simulink model "PrimRes_sharing"  (R2018a)
settings: Solver=VariableStepAuto  StartTime=0.0  StopTime=25  MaxStep=0.01  RelTol=1e-3
values from neighbouring files (symbols this model uses):
  Fn = 50    [PrimRes_sharing_Script.m]    (also in PrimRes_sharing_eigen_Script.m; PrimRes_sharing_steps_1_2MW_Script.m; PrimRes_sharing_steps_6MW_Script.m)
  KESS = Kess(4)    [PrimRes_sharing_Script.m]    (also in PrimRes_sharing_eigen_Script.m = Kess(i); PrimRes_sharing_steps_1_2MW_Script.m = Kess(i); PrimRes_sharing_steps_6MW_Script.m = Kess(i))
  KGT = Kgt(4)    [PrimRes_sharing_Script.m]    (also in PrimRes_sharing_eigen_Script.m = Kgt(i); PrimRes_sharing_steps_1_2MW_Script.m = Kgt(i); PrimRes_sharing_steps_6MW_Script.m = Kgt(i))
  Pessmax = 3    [PrimRes_sharing_Script.m]    (also in PrimRes_sharing_eigen_Script.m; PrimRes_sharing_steps_1_2MW_Script.m; PrimRes_sharing_steps_6MW_Script.m)
  Sn = 88    [PrimRes_sharing_Script.m]    (also in PrimRes_sharing_eigen_Script.m; PrimRes_sharing_steps_1_2MW_Script.m; PrimRes_sharing_steps_6MW_Script.m)
  StepMW = 6    [PrimRes_sharing_Script.m]    (also in PrimRes_sharing_eigen_Script.m = 1.2; PrimRes_sharing_steps_1_2MW_Script.m = 1.2; PrimRes_sharing_steps_6MW_Script.m)
  Tess = 0.05    [PrimRes_sharing_Script.m]    (also in PrimRes_sharing_eigen_Script.m; PrimRes_sharing_steps_1_2MW_Script.m; PrimRes_sharing_steps_6MW_Script.m)
  Tgov1 = 0.1    [PrimRes_sharing_Script.m]    (also in PrimRes_sharing_eigen_Script.m; PrimRes_sharing_steps_1_2MW_Script.m; PrimRes_sharing_steps_6MW_Script.m)
  Tgov2 = 0.4    [PrimRes_sharing_Script.m]    (also in PrimRes_sharing_eigen_Script.m; PrimRes_sharing_steps_1_2MW_Script.m; PrimRes_sharing_steps_6MW_Script.m)
settings Model: Creator=daniemot  LastModifiedBy=daniemot

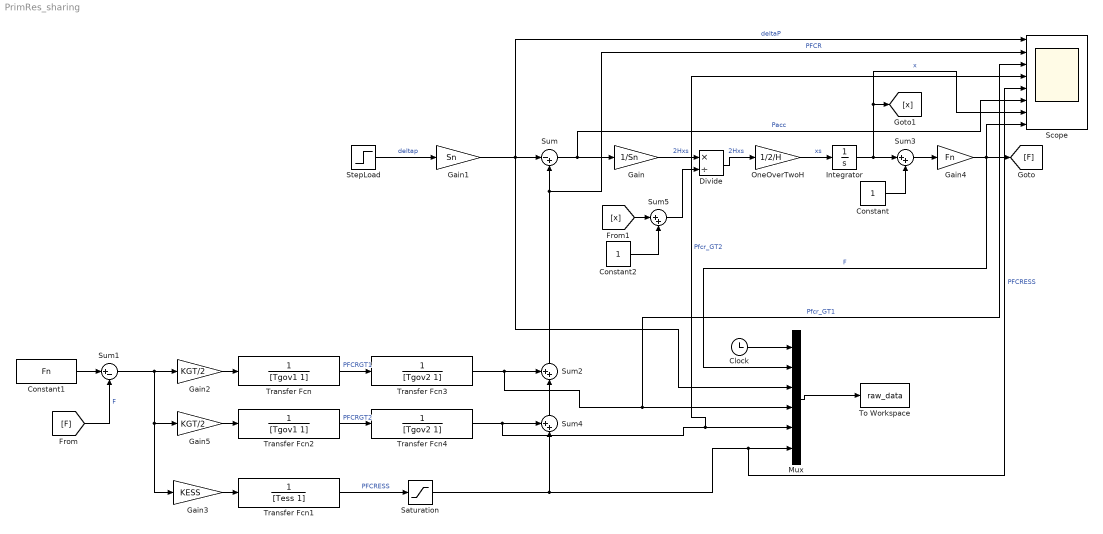
== system PrimRes_sharing ==
  Clock : Clock
  Constant : Constant
  Constant1 : Constant  Value=Fn
  Constant2 : Constant
  Divide : Product  Inputs=*/
  Gain : Gain  Gain=1/Sn
  Gain1 : Gain  Gain=Sn
  Gain2 : Gain  Gain=KGT/2
  Gain3 : Gain  Gain=KESS
  Gain4 : Gain  Gain=Fn
  Gain5 : Gain  Gain=KGT/2
  Integrator : Integrator
  Mux : Mux  Inputs=6
  OneOverTwoH : Gain  Gain=1/2/H
  Saturation : Saturate  UpperLimit=Pessmax  LowerLimit=-Pessmax
  Scope : Scope  NumInputPorts=8
  StepLoad : Step  After=StepMW/Sn  SampleTime=0
  Sum : Sum  Inputs=|-+
  Sum1 : Sum  Inputs=|+-
  Sum2 : Sum  Inputs=++|
  Sum3 : Sum  Inputs=|++
  Sum4 : Sum  Inputs=++|
  Sum5 : Sum  Inputs=|++
  To Workspace : ToWorkspace  VariableName=raw_data  SampleTime=-1
  Transfer Fcn : TransferFcn  Denominator=[Tgov1 1]
  Transfer Fcn1 : TransferFcn  Denominator=[Tess 1]
  Transfer Fcn2 : TransferFcn  Denominator=[Tgov1 1]
  Transfer Fcn3 : TransferFcn  Denominator=[Tgov2 1]
  Transfer Fcn4 : TransferFcn  Denominator=[Tgov2 1]
  wires:
  OneOverTwoH/1 -> Integrator/1  "xs"
  Divide/1 -> OneOverTwoH/1  "2Hxs"
  Sum/1 -> Scope/6, Gain/1  "Pacc"
  StepLoad/1 -> Gain1/1  "deltap"
  Integrator/1 -> Scope/7, [x], Sum3/1  "x"
  [F] -> Sum1/2  "F"
  Sum1/1 -> Gain2/1, Gain5/1, Gain3/1
  Constant1/1 -> Sum1/1
  Gain2/1 -> Transfer Fcn/1
  Sum2/1 -> Scope/2, Sum/2  "PFCR"
  Gain3/1 -> Transfer Fcn1/1
  Gain4/1 -> Scope/8, Mux/2, [F]  "F"
  Gain1/1 -> Mux/3, Scope/1, Sum/1  "deltaP"
  Sum3/1 -> Gain4/1
  Constant/1 -> Sum3/2
  Sum4/1 -> Sum2/2
  Gain5/1 -> Transfer Fcn2/1
  Transfer Fcn/1 -> Transfer Fcn3/1  "PFCRGT1"
  Transfer Fcn2/1 -> Transfer Fcn4/1  "PFCRGT2"
  Transfer Fcn3/1 -> Scope/3, Mux/4, Sum2/1  "Pfcr_GT1"
  Transfer Fcn4/1 -> Scope/4, Mux/5, Sum4/1  "Pfcr_GT2"
  Transfer Fcn1/1 -> Saturation/1  "PFCRESS"
  Mux/1 -> To Workspace/1
  Clock/1 -> Mux/1
  [x] -> Sum5/1
  Constant2/1 -> Sum5/2
  Gain/1 -> Divide/1  "2Hxs"
  Sum5/1 -> Divide/2
  Saturation/1 -> Scope/5, Mux/6, Sum4/2  "PFCRESS"
